simulink model "HWIL"  (R2025b)
settings: Solver=FixedStepAuto  StartTime=0.0  StopTime=10.0  FixedStep=1/1000  RelTol=1e-3
InitFcn:
  | plant_parameters;
undefined symbols (not defined in the file): mass
settings Model: Creator=karadeli  LastModifiedBy=karadeli
settings OptimizationCC: DefaultParameterBehavior=Inlined  UseDivisionForNetSlopeComputation=on  GainParamInheritBuiltInType=on  UseFloatMulNetSlope=on  InlineInvariantSignals=on  PassReuseOutputArgsAs=Individual arguments  ZeroExternalMemoryAtStartup=off  ZeroInternalMemoryAtStartup=off  NoFixptDivByZeroProtection=on  EfficientFloat2IntCast=on  LifeSpan=1  OptimizeBlockOrder=speed  DifferentSizesBufferReuse=on  EfficientTunableParamExpr=on
settings DebuggingCC: ParameterTunabilityLossMsg=error
settings HardwareCC: ProdBitPerPointer=32.0  ProdBitPerSizeT=32.0  ProdBitPerPtrDiffT=32.0  ProdLargestAtomicInteger=Long  ProdLargestAtomicFloat=Double  ProdWordSize=32.0  ProdLongLongMode=on  ProdHWDeviceType=ARM Compatible->ARM Cortex-M
settings SFSimCC: MATLABDynamicMemAlloc=off
settings RTWCC: SystemTargetFile=ert.tlc  GenCodeOnly=on  TemplateMakefile=ert_default_tmf  BuildConfiguration=Faster Runs  TargetLang=C++  Description=Embedded Coder
settings CodeAppCC: ForceParamTrailComments=on  IgnoreCustomStorageClasses=off  OperatorAnnotations=on  SimulinkDataObjDesc=on  SFDataObjDesc=on  CustomSymbolStrGlobalVar=rt$N$M  CustomSymbolStrType=$N$M  CustomSymbolStrFcn=$N$M$F  CustomSymbolStrMacro=$N$M  InsertBlockDesc=on
settings ERTTargetCC: RootIOFormat=Structure reference  ERTCustomFileTemplate=example_file_process.tlc  ERTFilePackagingFormat=CompactWithDataFile  TargetLangStandard=C++11 (ISO)  GenerateSampleERTMain=on  IncludeMdlTerminateFcn=off  CombineSignalStateStructs=on  SupportAbsoluteTime=off  CodeInterfacePackaging=C++ class  SubcomponentCodeInterfacePackaging=C++ class  SupportComplex=off  SupportContinuousTime=on

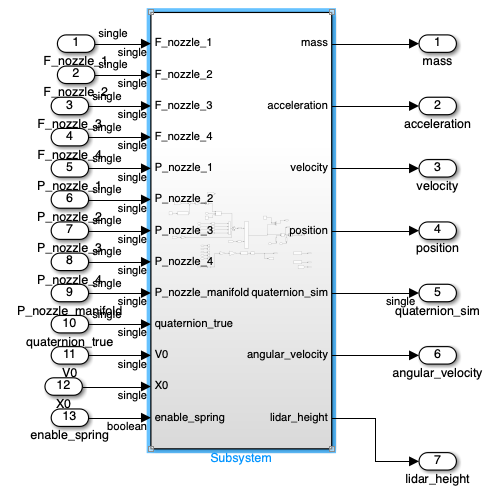
[thumbnail: Simulink's stored preview of the top-level diagram]
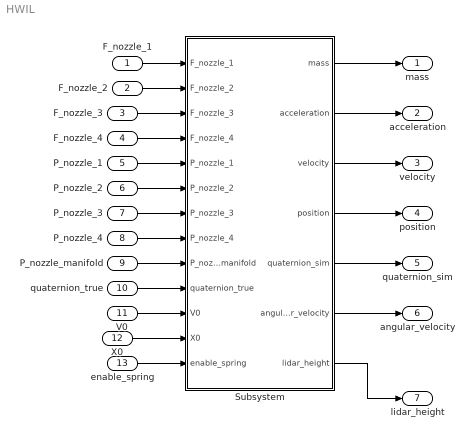
== system HWIL ==
  F_nozzle_1 : Inport  OutDataTypeStr=single  Unit=N
  F_nozzle_2 : Inport  Port=2  OutDataTypeStr=single  Unit=N
  F_nozzle_3 : Inport  Port=3  OutDataTypeStr=single  Unit=N
  F_nozzle_4 : Inport  Port=4  OutDataTypeStr=single  Unit=N
  P_nozzle_1 : Inport  Port=5  OutDataTypeStr=single  Unit=psi
  P_nozzle_2 : Inport  Port=6  OutDataTypeStr=single  Unit=psi
  P_nozzle_3 : Inport  Port=7  OutDataTypeStr=single  Unit=psi
  P_nozzle_4 : Inport  Port=8  OutDataTypeStr=single  Unit=psi
  P_nozzle_manifold : Inport  Port=9  OutDataTypeStr=single  Unit=psi
  quaternion_true : Inport  Port=10  OutDataTypeStr=single  PortDimensions=4
  V0 : Inport  Port=11
  X0 : Inport  Port=12
  enable_spring : Inport  Port=13
  Subsystem : Subsystem
  mass : Outport
  acceleration : Outport  Port=2  Unit=m/s^2
  velocity : Outport  Port=3
  position : Outport  Port=4
  quaternion_sim : Outport  Port=5  OutDataTypeStr=single  PortDimensions=4
  angular_velocity : Outport  Port=6  PortDimensions=3
  lidar_height : Outport  Port=7
  wires:
  F_nozzle_1/1 -> Subsystem/1(F_nozzle_1)
  F_nozzle_2/1 -> Subsystem/2(F_nozzle_2)
  F_nozzle_3/1 -> Subsystem/3(F_nozzle_3)
  F_nozzle_4/1 -> Subsystem/4(F_nozzle_4)
  P_nozzle_1/1 -> Subsystem/5(P_nozzle_1)
  P_nozzle_2/1 -> Subsystem/6(P_nozzle_2)
  P_nozzle_3/1 -> Subsystem/7(P_nozzle_3)
  P_nozzle_4/1 -> Subsystem/8(P_nozzle_4)
  P_nozzle_manifold/1 -> Subsystem/9(P_nozzle_manifold)
  quaternion_true/1 -> Subsystem/10(quaternion_true)
  Subsystem/1(mass) -> mass/1
  Subsystem/2(acceleration) -> acceleration/1
  Subsystem/3(velocity) -> velocity/1
  Subsystem/4(position) -> position/1
  V0/1 -> Subsystem/11(V0)
  X0/1 -> Subsystem/12(X0)
  enable_spring/1 -> Subsystem/13(enable_spring)
  Subsystem/5(quaternion_sim) -> quaternion_sim/1
  Subsystem/6(angular_velocity) -> angular_velocity/1
  Subsystem/7(lidar_height) -> lidar_height/1

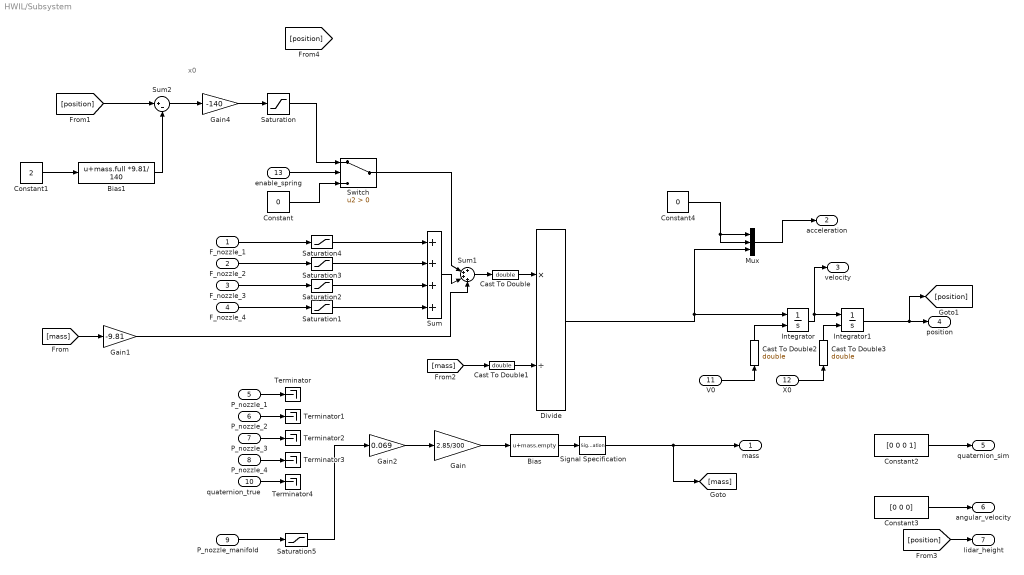
== system HWIL/Subsystem ==
  note: x0
  F_nozzle_1 : Inport  OutDataTypeStr=single  Unit=N
  F_nozzle_2 : Inport  Port=2  OutDataTypeStr=single  Unit=N
  F_nozzle_3 : Inport  Port=3  OutDataTypeStr=single  Unit=N
  F_nozzle_4 : Inport  Port=4  OutDataTypeStr=single  Unit=N
  P_nozzle_1 : Inport  Port=5  OutDataTypeStr=single  Unit=psi
  P_nozzle_2 : Inport  Port=6  OutDataTypeStr=single  Unit=psi
  P_nozzle_3 : Inport  Port=7  OutDataTypeStr=single  Unit=psi
  P_nozzle_4 : Inport  Port=8  OutDataTypeStr=single  Unit=psi
  P_nozzle_manifold : Inport  Port=9  OutDataTypeStr=single  Unit=psi  PortDimensions=1
  quaternion_true : Inport  Port=10  OutDataTypeStr=single  PortDimensions=4
  V0 : Inport  Port=11  OutDataTypeStr=single  Unit=m/s
  X0 : Inport  Port=12  OutDataTypeStr=single  Unit=m
  enable_spring : Inport  Port=13  OutDataTypeStr=boolean
  Bias : Bias  Bias=mass.empty  SaturateOnIntegerOverflow=off
  Bias1 : Bias  Bias=mass.full *9.81/ 140  SaturateOnIntegerOverflow=off
  Cast To Double{,1..3} (4 alike) : DataTypeConversion  OutDataTypeStr=double  SaturateOnIntegerOverflow=off  RndMeth=Floor
  Constant : Constant  Value=0
  Constant1 : Constant  Value=2
  Constant2 : Constant  Value=[0 0 0 1]  OutDataTypeStr=single
  Constant3 : Constant  Value=[0 0 0]  OutDataTypeStr=single
  Constant4 : Constant  Value=0
  Divide : Product  Inputs=*/
  Gain : Gain  Gain=2.85/300
  Gain1 : Gain  Gain=-9.81
  Gain2 : Gain  Gain=0.069
  Gain4 : Gain  Gain=-140
  Integrator : Integrator  InitialConditionSource=external
  Integrator1 : Integrator  InitialConditionSource=external  LimitOutput=on  LowerSaturationLimit=0
  Mux : Mux  Inputs=3
  Saturation : Saturate  UpperLimit=(35*9.81/140+2)*140  LowerLimit=0
  Saturation{1..5} (5 alike) : Saturate  UpperLimit=inf  LowerLimit=0
  Signal Specification : SignalSpecification  Unit=kg
  Sum : Sum  Inputs=4
  Sum1 : Sum  Inputs=4
  Sum2 : Sum  Inputs=|+-
  Switch : Switch  Criteria=u2 > Threshold  SaturateOnIntegerOverflow=off  InputSameDT=off
  Terminator{,1..4} (5 alike) : Terminator
  mass : Outport  Unit=kg
  acceleration : Outport  Port=2  Unit=m/s^2
  velocity : Outport  Port=3  Unit=m/s
  position : Outport  Port=4  Unit=m
  quaternion_sim : Outport  Port=5
  angular_velocity : Outport  Port=6
  lidar_height : Outport  Port=7
  wires:
  F_nozzle_4/1 -> Saturation1/1
  F_nozzle_3/1 -> Saturation2/1
  F_nozzle_2/1 -> Saturation3/1
  F_nozzle_1/1 -> Saturation4/1
  Bias/1 -> Signal Specification/1
  P_nozzle_manifold/1 -> Saturation5/1
  Signal Specification/1 -> [mass], mass/1
  Gain/1 -> Bias/1
  Sum/1 -> Sum1/3
  [mass] -> Gain1/1
  Gain1/1 -> Sum1/4
  Sum1/1 -> Cast To Double/1
  [mass] -> Cast To Double1/1
  Divide/1 -> Mux/3, Integrator/1
  Integrator/1 -> Integrator1/1, velocity/1
  Integrator1/1 -> [position], position/1
  P_nozzle_1/1 -> Terminator/1
  P_nozzle_2/1 -> Terminator1/1
  P_nozzle_3/1 -> Terminator2/1
  P_nozzle_4/1 -> Terminator3/1
  quaternion_true/1 -> Terminator4/1
  V0/1 -> Cast To Double2/1
  X0/1 -> Cast To Double3/1
  Cast To Double/1 -> Divide/1
  Cast To Double1/1 -> Divide/2
  Cast To Double2/1 -> Integrator/2
  Cast To Double3/1 -> Integrator1/2
  Gain2/1 -> Gain/1
  Switch/1 -> Sum1/2
  enable_spring/1 -> Switch/2
  Constant/1 -> Switch/3
  Constant1/1 -> Bias1/1
  [position] -> Sum2/1
  Sum2/1 -> Gain4/1
  Gain4/1 -> Saturation/1
  Bias1/1 -> Sum2/2
  Saturation/1 -> Switch/1
  Constant2/1 -> quaternion_sim/1
  Constant3/1 -> angular_velocity/1
  Constant4/1 -> Mux/2, Mux/1
  Mux/1 -> acceleration/1
  [position] -> lidar_height/1
  Saturation1/1 -> Sum/4
  Saturation2/1 -> Sum/3
  Saturation3/1 -> Sum/2
  Saturation4/1 -> Sum/1
  Saturation5/1 -> Gain2/1
